simulink model "SimulationTest"  (R2024a)
settings: Solver=ode8  StartTime=0.0  StopTime=1000  FixedStep=0.1  RelTol=1e-3
model workspace (MAT data in the model file):
  L = 0.25
  R = 0.05
libraries: simulink x2
settings Model: PacingRate=1000  Creator=levirogalla  LastModifiedBy=levirogalla

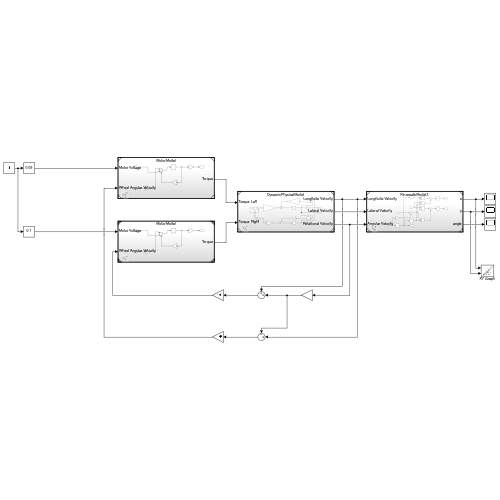
[thumbnail: Simulink's stored preview of the top-level diagram]
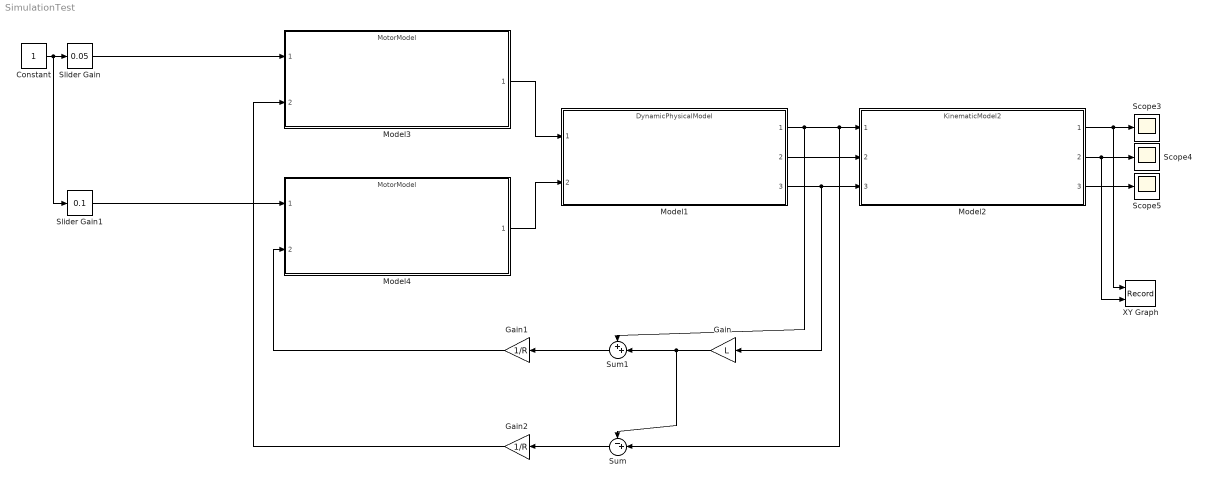
== system SimulationTest ==
  Constant : Constant
  Gain : Gain  Gain=L
  Gain1 : Gain  Gain=1/R
  Gain2 : Gain  Gain=1/R
  Model1 : ModelReference  ModelNameDialog=DynamicPhysicalModel.slx  SimulationMode=Normal  ModelReferenceVersion=1.6
  Model2 : ModelReference  ModelNameDialog=KinematicModel2.slx  SimulationMode=Normal  ModelReferenceVersion=1.4
  Model3 : ModelReference  ModelNameDialog=MotorModel.slx  SimulationMode=Normal  ModelReferenceVersion=1.4
  Model4 : ModelReference  ModelNameDialog=MotorModel.slx  SimulationMode=Normal  ModelReferenceVersion=1.4
  Scope3 : Scope
  Scope4 : Scope
  Scope5 : Scope
  Slider Gain : simulink/Math Operations/Slider Gain  gain=0.05  low=-1  high=1
  Slider Gain1 : simulink/Math Operations/Slider Gain  gain=0.1  low=-1  high=1
  Sum : Sum  Inputs=-+|
  Sum1 : Sum  Inputs=++|
  XY Graph : Record  FileSettingsInternal="{\"entries\":[{\"content\":{\"excelSettings\":{\"content\":{},\"type\":\"Streamout.ExcelSettings\"}},\"type\":\"Streamout.FileSettingStorage\",\"uuid\":\"\"}],\"packageUris\":[\"http:\\/\\/schema.mathworks.com\\/mf0\\/streamout_blocks\\/R2020a\"],\"version\":\"1.0\"}"  Layout=[1 1]  SignalsInternal="{\"entries\":[{\"content\":{\"signals\":[{\"content\":{\"blockPath\":[],\"dimensions\":[1],\"domain\":\"\",\"lineColor\":\"#a2142f\",\"plots\":[ 1 ],\"port\":1,\"sid\":[\"\"],\"signalID\":1,\"signalName\":\"Model2:1\"},\"type\":\"RecordBlkView.Signal\",\"uuid\":\"\"},{\"content\":{\"blockPath\":[],\"dimensions\":[1],\"domain\":\"\",\"lineColor\":\"#139fff\",\"plots\":[ 1 ],\"port\":2,\"sid\":[\"\"],\"signalID\":2,\"signalName\":\"Model2:2\"},\"type\":\"RecordBlkView.Signal\",\"uuid\":\"\"}]},\"type\":\"RecordBlkView.InputSignals\",\"uuid\":\"\"}],\"packageUris\":[\"http:\\/\\/schema.mathworks.com\\/mf0\\/streamout_blocks\\/R2020a\"],\"version\":\"1.0\"}"  VisualizationBindings="{\"xyplotplugin\":{\"info\":[{\"series\":[{\"bindingParametersList\":[{\"parameter\":\"X-Axis\",\"signalID\":1,\"signalName\":\"Model2:1\"},{\"parameter\":\"Y-Axis\",\"signalID\":2,\"signalName\":\"Model2:2\"}],\"seriesID\":0}],\"subplotID\":1}]}}"  CompatibilityTag=XY
  wires:
  Model1/3 -> Gain/1, Model2/3
  Model1/2 -> Model2/2
  Model1/1 -> Sum1/1, Sum/2, Model2/1
  Model2/1 -> XY Graph/1, Scope3/1
  Model2/2 -> XY Graph/2, Scope4/1
  Model2/3 -> Scope5/1
  Constant/1 -> Slider Gain1/1, Slider Gain/1
  Model4/1 -> Model1/2
  Model3/1 -> Model1/1
  Slider Gain/1 -> Model3/1
  Slider Gain1/1 -> Model4/1
  Gain/1 -> Sum/1, Sum1/2
  Sum1/1 -> Gain1/1
  Sum/1 -> Gain2/1
  Gain1/1 -> Model4/2
  Gain2/1 -> Model3/2
